simulink model "file2"  (R2025b)
settings: Solver=VariableStepAuto  StartTime=0.0  StopTime=1.0  RelTol=1e-3
InitFcn:
  | Voc= 32.9;
  | Iscn = 8.21;
  | K=1.38e-23;
  | N5=54;
  | Np=1;
  | G1 = 1000;
  | G2 = 859;
  | G3 = 659;
  | Gn = 1000;
  | Kv= - 0.123;
  | K1=0.0032;
  | T=301;
  | Tn = 300;
  | q=1.6e-19;
  | I0n = 9.58e-8;
  | Eg =1.12;
  | Ign =8.214;
  | Rs = 0.221;
  | Rp =414.5;
  | a=1.0;
libraries: spsVoltageMeasurementLib x7, spsSeriesRLCBranchLib x6, spsDiodeLib x3, spsControlledCurrentSourceLib x3, spsControlledVoltageSourceLib x1, spsCurrentMeasurementLib x1, simulink x1, spspowerguiLib x1
settings Model: Creator=cdsl09  LastModifiedBy=hp

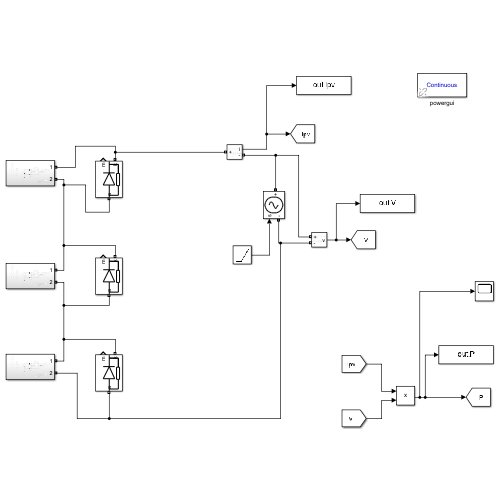
[thumbnail: Simulink's stored preview of the top-level diagram]
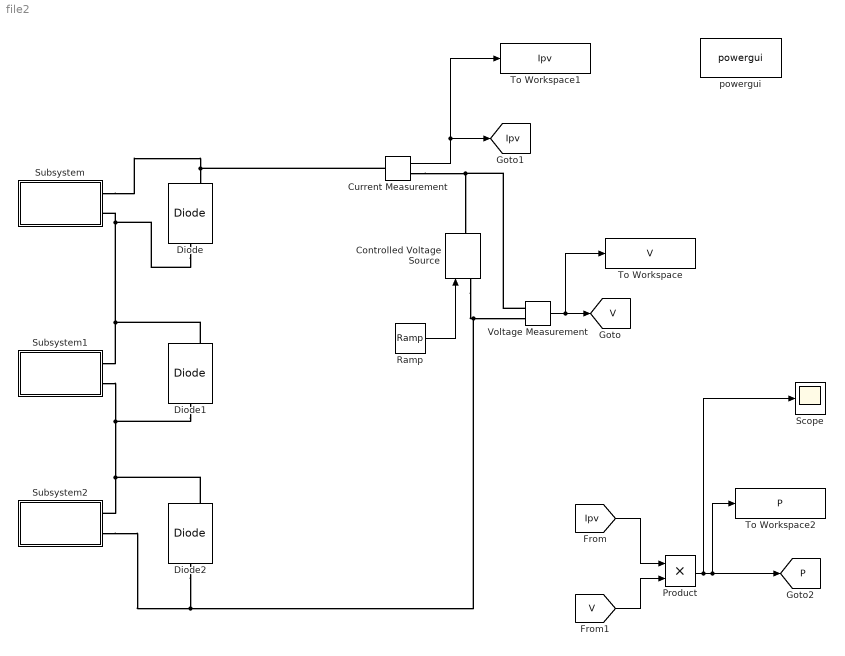
== system file2 ==
  Controlled Voltage Source : spsControlledVoltageSourceLib/Controlled Voltage Source  Initialize=on  Source_Type=AC  Amplitude=0  Phase=0  Frequency=0  Measurements=None
  Current Measurement : spsCurrentMeasurementLib/Current Measurement  PhasorSimulation=off  OutputType=Complex  PSBequivalent=0
  Diode : spsDiodeLib/Diode  Ron=0.001  Lon=0  Vf=0.8  IC=0  UseSnubber=0  Rs=500  Cs=250e-9  Measurements=on
  Diode1 : spsDiodeLib/Diode  Ron=0.001  Lon=0  Vf=0.8  IC=0  UseSnubber=0  Rs=500  Cs=250e-9  Measurements=on
  Diode2 : spsDiodeLib/Diode  Ron=0.001  Lon=0  Vf=0.8  IC=0  UseSnubber=0  Rs=500  Cs=250e-9  Measurements=on
  Product : Product
  Ramp : simulink/Sources/Ramp  slope=100  start=0  InitialOutput=0
  Scope : Scope
      settings: ActiveDisplayYMinimum=-293.34579  ActiveDisplayYMaximum=493.69358
  Subsystem : Subsystem
  Subsystem1 : Subsystem
  Subsystem2 : Subsystem
  To Workspace : ToWorkspace  VariableName=V  SampleTime=-1
  To Workspace1 : ToWorkspace  VariableName=Ipv  SampleTime=-1
  To Workspace2 : ToWorkspace  VariableName=P  SampleTime=-1
  Voltage Measurement : spsVoltageMeasurementLib/Voltage Measurement  PhasorSimulation=off  OutputType=Complex  PSBequivalent=0
  powergui : spspowerguiLib/powergui  Priority=1  SimulationMode=Continuous  SampleTime=50e-6  frequency=60  Iterations=50  frequencyindice=0  Pbase=100e6  ErrMax=1e-4  UnitsV=kV  UnitsW=MW  buscounter=0  FunctionMessages=off  echomessages=off  EnableUseOfTLC=off  CurrentSourceSwitches=off  DisableSnubberDevices=off  DisableRonSwitches=off  DisableVfSwitches=off  DisplayEquations=off  AutomaticDiscreteSolvers=off  SolverType=Tustin/Backward Euler (TBE)  Interpol=off  ExternalGateDelay=off  methode=off  Ts=100  x0status=blocks  SPID=on  SwTol=0  HookPort=off  NonlinearTolerance=1e-4  nMaxIteration=100  ContinueOnMaxIteration=off  RestoreLinks=warning  ResistiveCurrentMeasurement=off  Frange=[0:2:500]  Ylog=off  Xlog=on  ShowGrid=off  save=off  variable=ZData  structure=0  ZoomFFT=off  StartTime=0.0  cycles=1  DisplayStyle=1  fundamental=60  FreqAxis=off  MaxFrequency=1000  frequencyindicesteady=1  RmsSteady=1  display=off
  tag scope: Ipv=global, P=global, V=global
  wires:
  Ramp/1 -> Controlled Voltage Source/1
  Voltage Measurement/1 -> To Workspace/1, [V]
  Current Measurement/1 -> To Workspace1/1, [Ipv]
  [Ipv] -> Product/1
  [V] -> Product/2
  Product/1 -> Scope/1, To Workspace2/1, [P]
  connections:
  Subsystem/LConn1 -- Current Measurement/LConn1 -- Diode/RConn1
  Subsystem1/LConn1 -- Diode1/RConn1 -- Diode/LConn1 -- Subsystem/LConn2
  Subsystem1/LConn2 -- Diode1/LConn1 -- Diode2/RConn1 -- Subsystem2/LConn1
  Current Measurement/RConn1 -- Voltage Measurement/LConn1 -- Controlled Voltage Source/RConn1
  Controlled Voltage Source/LConn1 -- Diode2/LConn1 -- Subsystem2/LConn2 -- Voltage Measurement/LConn2

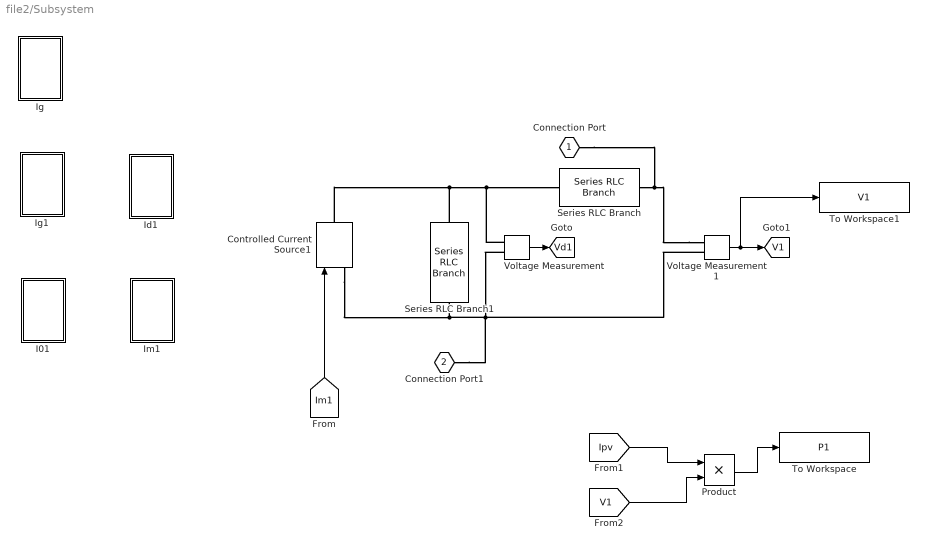
== system file2/Subsystem ==
  Controlled Current Source1 : spsControlledCurrentSourceLib/Controlled Current Source  Initialize=on  Source_Type=AC  Amplitude=0  Phase=0  Frequency=0  Measurements=None
  I01 : Subsystem
  Id1 : Subsystem
  Ig : Subsystem
  Ig1 : Subsystem
  Im1 : Subsystem
  Product : Product
  Series RLC Branch : spsSeriesRLCBranchLib/Series RLC Branch  LConnTagsString=__new0  RConnTagsString=__new0  BranchType=R  Resistance=Rs  Inductance=1e-3  SetiL0=off  InitialCurrent=0  Capacitance=1e-6  Setx0=off  InitialVoltage=0  Measurements=None
  Series RLC Branch1 : spsSeriesRLCBranchLib/Series RLC Branch  LConnTagsString=__new0  RConnTagsString=__new0  BranchType=R  Resistance=Rp  Inductance=1e-3  SetiL0=off  InitialCurrent=0  Capacitance=1e-6  Setx0=off  InitialVoltage=0  Measurements=None
  To Workspace : ToWorkspace  VariableName=P1  SaveFormat=Timeseries  SampleTime=-1
  To Workspace1 : ToWorkspace  VariableName=V1  SaveFormat=Timeseries  SampleTime=-1
  Voltage Measurement : spsVoltageMeasurementLib/Voltage Measurement  PhasorSimulation=off  OutputType=Complex  PSBequivalent=0
  Voltage Measurement1 : spsVoltageMeasurementLib/Voltage Measurement  PhasorSimulation=off  OutputType=Complex  PSBequivalent=0
  Connection Port : PMIOPort  Tag=simrfV2util1/Connection Port  Side=Left
  Connection Port1 : PMIOPort  Tag=simrfV2util1/Connection Port  Port=2  Side=Left
  tag scope: V1=global, Vd1=global
  wires:
  Product/1 -> To Workspace/1
  Voltage Measurement/1 -> [Vd1]
  Voltage Measurement1/1 -> To Workspace1/1, [V1]
  [Ipv] -> Product/1
  [Im1] -> Controlled Current Source1/1
  [V1] -> Product/2
  connections:
  Controlled Current Source1/LConn1 -- Connection Port1/RConn1 -- Voltage Measurement1/LConn2 -- Voltage Measurement/LConn2 -- Series RLC Branch1/LConn1
  Controlled Current Source1/RConn1 -- Series RLC Branch1/RConn1 -- Voltage Measurement/LConn1 -- Series RLC Branch/LConn1
  Voltage Measurement1/LConn1 -- Connection Port/RConn1 -- Series RLC Branch/RConn1

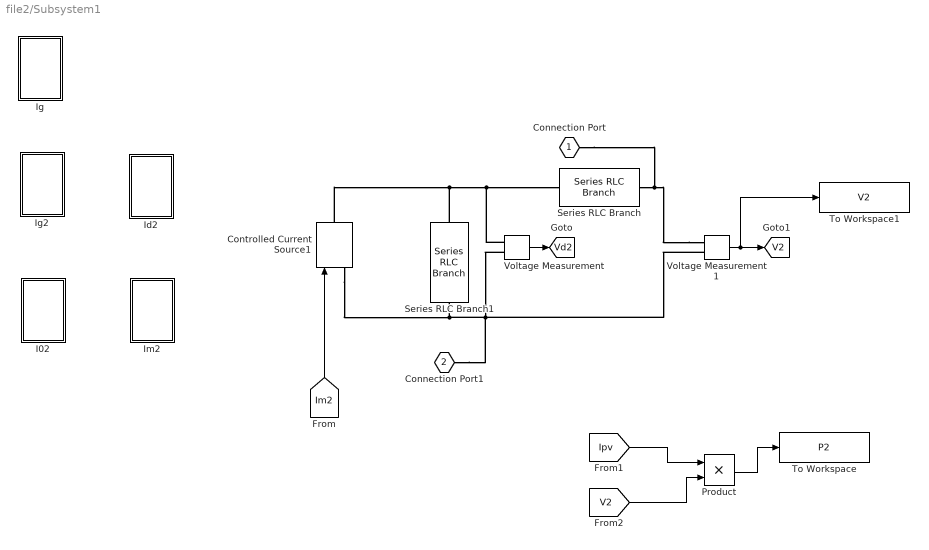
== system file2/Subsystem1 ==
  Controlled Current Source1 : spsControlledCurrentSourceLib/Controlled Current Source  Initialize=on  Source_Type=AC  Amplitude=0  Phase=0  Frequency=0  Measurements=None
  I02 : Subsystem
  Id2 : Subsystem
  Ig : Subsystem
  Ig2 : Subsystem
  Im2 : Subsystem
  Product : Product
  Series RLC Branch : spsSeriesRLCBranchLib/Series RLC Branch  LConnTagsString=__new0  RConnTagsString=__new0  BranchType=R  Resistance=Rs  Inductance=1e-3  SetiL0=off  InitialCurrent=0  Capacitance=1e-6  Setx0=off  InitialVoltage=0  Measurements=None
  Series RLC Branch1 : spsSeriesRLCBranchLib/Series RLC Branch  LConnTagsString=__new0  RConnTagsString=__new0  BranchType=R  Resistance=Rp  Inductance=1e-3  SetiL0=off  InitialCurrent=0  Capacitance=1e-6  Setx0=off  InitialVoltage=0  Measurements=None
  To Workspace : ToWorkspace  VariableName=P2  SaveFormat=Timeseries  SampleTime=-1
  To Workspace1 : ToWorkspace  VariableName=V2  SaveFormat=Timeseries  SampleTime=-1
  Voltage Measurement : spsVoltageMeasurementLib/Voltage Measurement  PhasorSimulation=off  OutputType=Complex  PSBequivalent=0
  Voltage Measurement1 : spsVoltageMeasurementLib/Voltage Measurement  PhasorSimulation=off  OutputType=Complex  PSBequivalent=0
  Connection Port : PMIOPort  Tag=simrfV2util1/Connection Port  Side=Left
  Connection Port1 : PMIOPort  Tag=simrfV2util1/Connection Port  Port=2  Side=Left
  tag scope: V2=global, Vd2=global
  wires:
  Product/1 -> To Workspace/1
  Voltage Measurement/1 -> [Vd2]
  Voltage Measurement1/1 -> To Workspace1/1, [V2]
  [Ipv] -> Product/1
  [Im2] -> Controlled Current Source1/1
  [V2] -> Product/2
  connections:
  Controlled Current Source1/LConn1 -- Series RLC Branch1/LConn1 -- Voltage Measurement1/LConn2 -- Voltage Measurement/LConn2 -- Connection Port1/RConn1
  Controlled Current Source1/RConn1 -- Series RLC Branch1/RConn1 -- Voltage Measurement/LConn1 -- Series RLC Branch/LConn1
  Voltage Measurement1/LConn1 -- Series RLC Branch/RConn1 -- Connection Port/RConn1

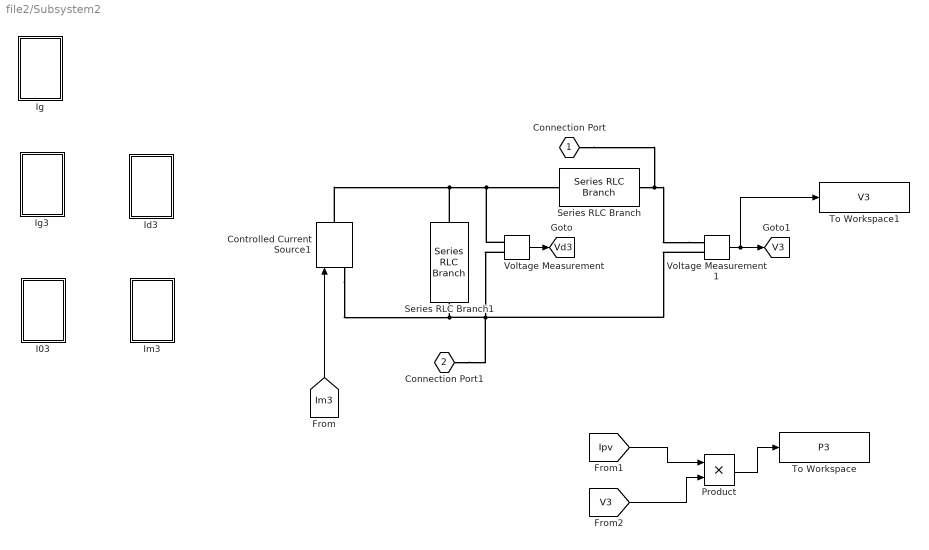
== system file2/Subsystem2 ==
  Controlled Current Source1 : spsControlledCurrentSourceLib/Controlled Current Source  Initialize=on  Source_Type=AC  Amplitude=0  Phase=0  Frequency=0  Measurements=None
  I03 : Subsystem
  Id3 : Subsystem
  Ig : Subsystem
  Ig3 : Subsystem
  Im3 : Subsystem
  Product : Product
  Series RLC Branch : spsSeriesRLCBranchLib/Series RLC Branch  LConnTagsString=__new0  RConnTagsString=__new0  BranchType=R  Resistance=Rs  Inductance=1e-3  SetiL0=off  InitialCurrent=0  Capacitance=1e-6  Setx0=off  InitialVoltage=0  Measurements=None
  Series RLC Branch1 : spsSeriesRLCBranchLib/Series RLC Branch  LConnTagsString=__new0  RConnTagsString=__new0  BranchType=R  Resistance=Rp  Inductance=1e-3  SetiL0=off  InitialCurrent=0  Capacitance=1e-6  Setx0=off  InitialVoltage=0  Measurements=None
  To Workspace : ToWorkspace  VariableName=P3  SaveFormat=Timeseries  SampleTime=-1
  To Workspace1 : ToWorkspace  VariableName=V3  SaveFormat=Timeseries  SampleTime=-1
  Voltage Measurement : spsVoltageMeasurementLib/Voltage Measurement  PhasorSimulation=off  OutputType=Complex  PSBequivalent=0
  Voltage Measurement1 : spsVoltageMeasurementLib/Voltage Measurement  PhasorSimulation=off  OutputType=Complex  PSBequivalent=0
  Connection Port : PMIOPort  Tag=simrfV2util1/Connection Port  Side=Left
  Connection Port1 : PMIOPort  Tag=simrfV2util1/Connection Port  Port=2  Side=Left
  tag scope: V3=global, Vd3=global
  wires:
  Product/1 -> To Workspace/1
  Voltage Measurement/1 -> [Vd3]
  Voltage Measurement1/1 -> To Workspace1/1, [V3]
  [Ipv] -> Product/1
  [Im3] -> Controlled Current Source1/1
  [V3] -> Product/2
  connections:
  Controlled Current Source1/LConn1 -- Series RLC Branch1/LConn1 -- Voltage Measurement1/LConn2 -- Voltage Measurement/LConn2 -- Connection Port1/RConn1
  Controlled Current Source1/RConn1 -- Series RLC Branch1/RConn1 -- Voltage Measurement/LConn1 -- Series RLC Branch/LConn1
  Voltage Measurement1/LConn1 -- Series RLC Branch/RConn1 -- Connection Port/RConn1

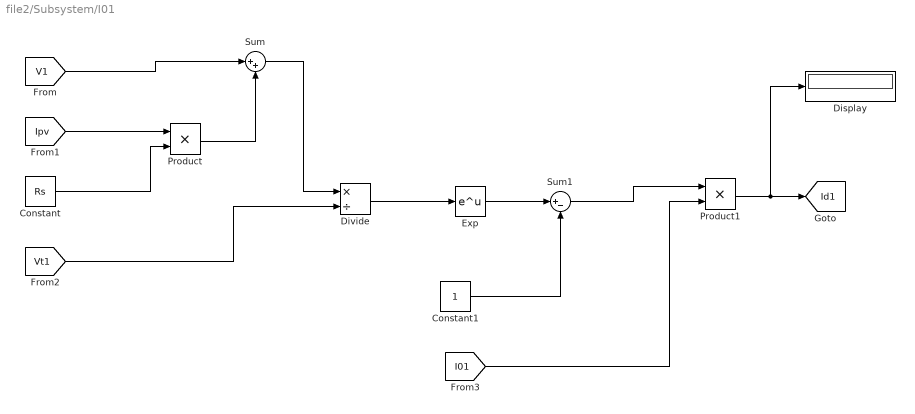
== system file2/Subsystem/I01 ==
  Constant : Constant  Value=Rs
  Constant1 : Constant
  Display : Display
  Divide : Product  Inputs=*/
  Exp : Math
  Product : Product
  Product1 : Product
  Sum : Sum  Inputs=|++
  Sum1 : Sum  Inputs=|+-
  tag scope: Id1=global
  wires:
  Exp/1 -> Sum1/1
  Divide/1 -> Exp/1
  [I01] -> Product1/2
  Sum/1 -> Divide/1
  [V1] -> Sum/1
  Product/1 -> Sum/2
  Constant1/1 -> Sum1/2
  Sum1/1 -> Product1/1
  Constant/1 -> Product/2
  [Ipv] -> Product/1
  [Vt1] -> Divide/2
  Product1/1 -> Display/1, [Id1]

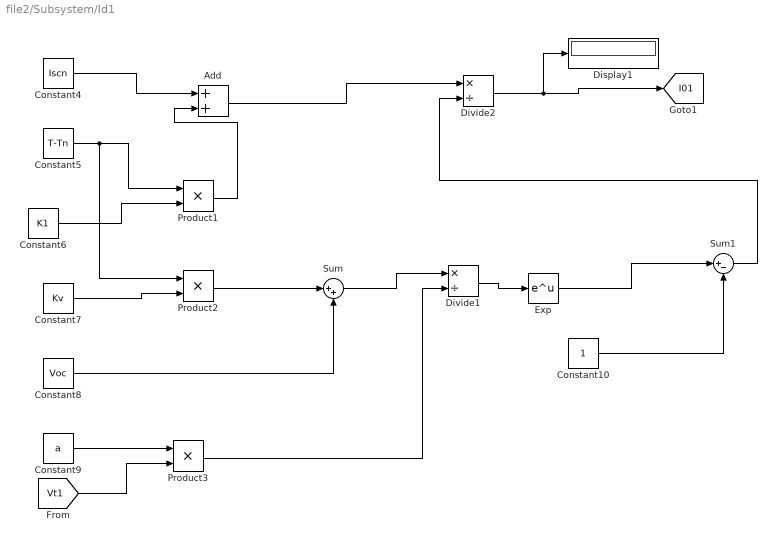
== system file2/Subsystem/Id1 ==
  Add : Sum
  Constant10 : Constant
  Constant4 : Constant  Value=Iscn
  Constant5 : Constant  Value=T-Tn
  Constant6 : Constant  Value=K1
  Constant7 : Constant  Value=Kv
  Constant8 : Constant  Value=Voc
  Constant9 : Constant  Value=a
  Display1 : Display
  Divide1 : Product  Inputs=*/
  Divide2 : Product  Inputs=*/
  Exp : Math
  Product1 : Product
  Product2 : Product
  Product3 : Product
  Sum : Sum  Inputs=|++
  Sum1 : Sum  Inputs=|+-
  tag scope: I01=global
  wires:
  Product2/1 -> Sum/1
  Constant8/1 -> Sum/2
  Constant4/1 -> Add/1
  Constant5/1 -> Product2/1, Product1/1
  Product1/1 -> Add/2
  Product3/1 -> Divide1/2
  Divide1/1 -> Exp/1
  Constant6/1 -> Product1/2
  Sum1/1 -> Divide2/2
  [Vt1] -> Product3/2
  Constant9/1 -> Product3/1
  Divide2/1 -> Display1/1, [I01]
  Constant10/1 -> Sum1/2
  Add/1 -> Divide2/1
  Constant7/1 -> Product2/2
  Exp/1 -> Sum1/1
  Sum/1 -> Divide1/1

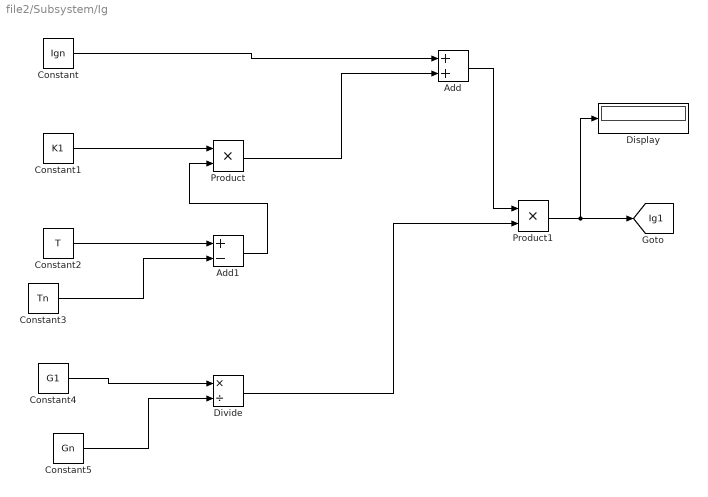
== system file2/Subsystem/Ig ==
  Add : Sum
  Add1 : Sum  Inputs=+-
  Constant : Constant  Value=Ign
  Constant1 : Constant  Value=K1
  Constant2 : Constant  Value=T
  Constant3 : Constant  Value=Tn
  Constant4 : Constant  Value=G1  VectorParams1D=off
  Constant5 : Constant  Value=Gn
  Display : Display
  Divide : Product  Inputs=*/
  Product : Product
  Product1 : Product
  tag scope: Ig1=global
  wires:
  Product1/1 -> Display/1, [Ig1]
  Constant3/1 -> Add1/2
  Constant5/1 -> Divide/2
  Add1/1 -> Product/2
  Constant4/1 -> Divide/1
  Product/1 -> Add/2
  Constant2/1 -> Add1/1
  Add/1 -> Product1/1
  Constant1/1 -> Product/1
  Constant/1 -> Add/1
  Divide/1 -> Product1/2

== system file2/Subsystem/Ig1 ==
  Constant : Constant  Value=N5
  Constant1 : Constant  Value=K
  Constant2 : Constant  Value=T
  Constant3 : Constant  Value=q
  Display : Display
  Divide : Product  Inputs=*/
  Product : Product  Inputs=3
  tag scope: Vt1=global
  wires:
  Product/1 -> Divide/1
  Constant/1 -> Product/1
  Constant3/1 -> Divide/2
  Constant1/1 -> Product/2
  Constant2/1 -> Product/3
  Divide/1 -> Display/1, [Vt1]

== system file2/Subsystem/Im1 ==
  Add : Sum  Inputs=+-
  Display : Display
  tag scope: Im1=global
  wires:
  [Ig1] -> Add/1
  [Id1] -> Add/2
  Add/1 -> Display/1, [Im1]

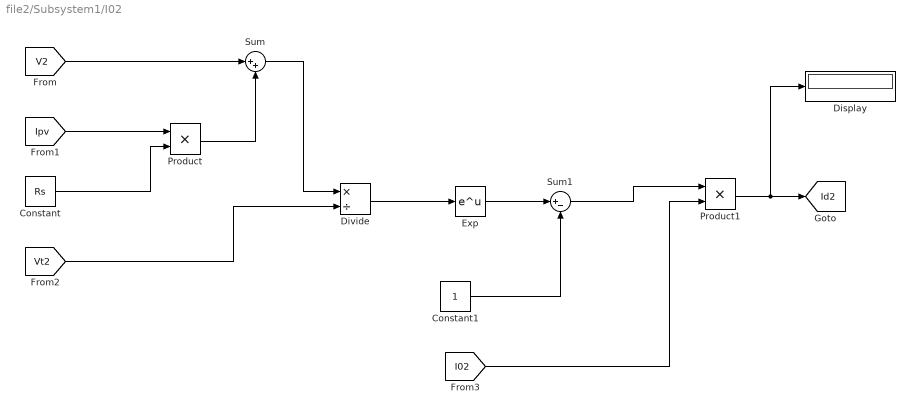
== system file2/Subsystem1/I02 ==
  Constant : Constant  Value=Rs
  Constant1 : Constant
  Display : Display
  Divide : Product  Inputs=*/
  Exp : Math
  Product : Product
  Product1 : Product
  Sum : Sum  Inputs=|++
  Sum1 : Sum  Inputs=|+-
  tag scope: Id2=global
  wires:
  Exp/1 -> Sum1/1
  Divide/1 -> Exp/1
  [I02] -> Product1/2
  Sum/1 -> Divide/1
  [V2] -> Sum/1
  Product/1 -> Sum/2
  Constant1/1 -> Sum1/2
  Sum1/1 -> Product1/1
  Constant/1 -> Product/2
  [Ipv] -> Product/1
  [Vt2] -> Divide/2
  Product1/1 -> Display/1, [Id2]

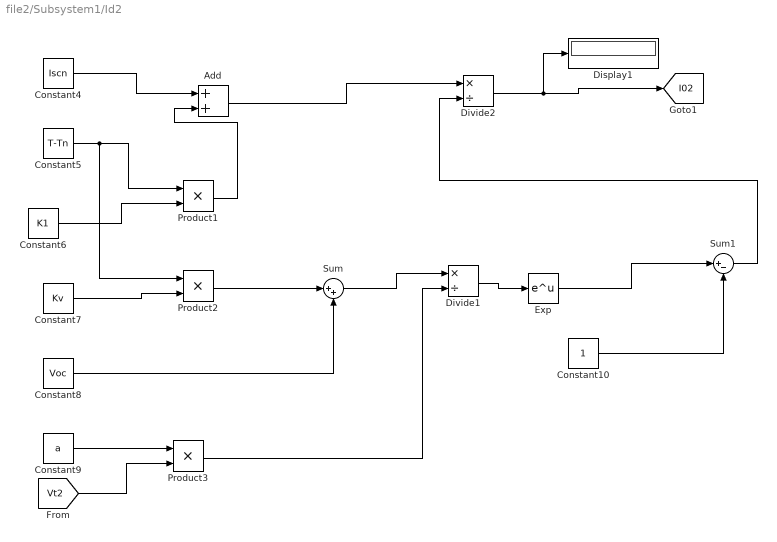
== system file2/Subsystem1/Id2 ==
  Add : Sum
  Constant10 : Constant
  Constant4 : Constant  Value=Iscn
  Constant5 : Constant  Value=T-Tn
  Constant6 : Constant  Value=K1
  Constant7 : Constant  Value=Kv
  Constant8 : Constant  Value=Voc
  Constant9 : Constant  Value=a
  Display1 : Display
  Divide1 : Product  Inputs=*/
  Divide2 : Product  Inputs=*/
  Exp : Math
  Product1 : Product
  Product2 : Product
  Product3 : Product
  Sum : Sum  Inputs=|++
  Sum1 : Sum  Inputs=|+-
  tag scope: I02=global
  wires:
  Product2/1 -> Sum/1
  Constant8/1 -> Sum/2
  Constant4/1 -> Add/1
  Constant5/1 -> Product2/1, Product1/1
  Product1/1 -> Add/2
  Product3/1 -> Divide1/2
  Divide1/1 -> Exp/1
  Constant6/1 -> Product1/2
  Sum1/1 -> Divide2/2
  [Vt2] -> Product3/2
  Constant9/1 -> Product3/1
  Divide2/1 -> Display1/1, [I02]
  Constant10/1 -> Sum1/2
  Add/1 -> Divide2/1
  Constant7/1 -> Product2/2
  Exp/1 -> Sum1/1
  Sum/1 -> Divide1/1

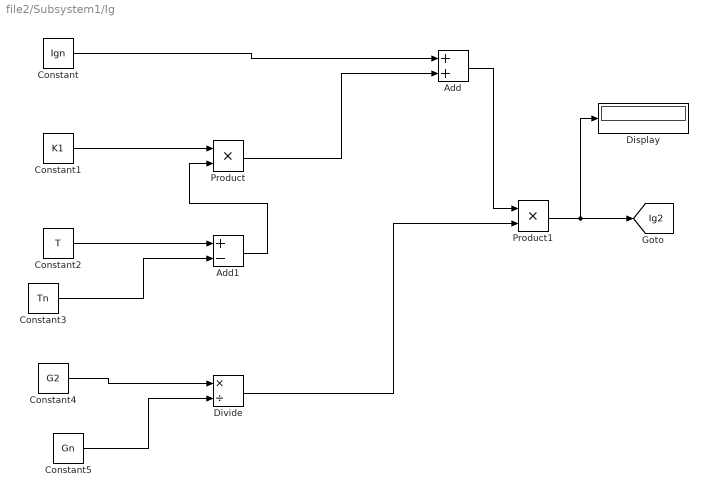
== system file2/Subsystem1/Ig ==
  Add : Sum
  Add1 : Sum  Inputs=+-
  Constant : Constant  Value=Ign
  Constant1 : Constant  Value=K1
  Constant2 : Constant  Value=T
  Constant3 : Constant  Value=Tn
  Constant4 : Constant  Value=G2  VectorParams1D=off
  Constant5 : Constant  Value=Gn
  Display : Display
  Divide : Product  Inputs=*/
  Product : Product
  Product1 : Product
  tag scope: Ig2=global
  wires:
  Product1/1 -> Display/1, [Ig2]
  Constant3/1 -> Add1/2
  Constant5/1 -> Divide/2
  Add1/1 -> Product/2
  Constant4/1 -> Divide/1
  Product/1 -> Add/2
  Constant2/1 -> Add1/1
  Add/1 -> Product1/1
  Constant1/1 -> Product/1
  Constant/1 -> Add/1
  Divide/1 -> Product1/2

== system file2/Subsystem1/Ig2 ==
  Constant : Constant  Value=N5
  Constant1 : Constant  Value=K
  Constant2 : Constant  Value=T
  Constant3 : Constant  Value=q
  Display : Display
  Divide : Product  Inputs=*/
  Product : Product  Inputs=3
  tag scope: Vt2=global
  wires:
  Product/1 -> Divide/1
  Constant/1 -> Product/1
  Constant3/1 -> Divide/2
  Constant1/1 -> Product/2
  Constant2/1 -> Product/3
  Divide/1 -> Display/1, [Vt2]

== system file2/Subsystem1/Im2 ==
  Add : Sum  Inputs=+-
  Display : Display
  tag scope: Im2=global
  wires:
  [Ig2] -> Add/1
  [Id2] -> Add/2
  Add/1 -> Display/1, [Im2]

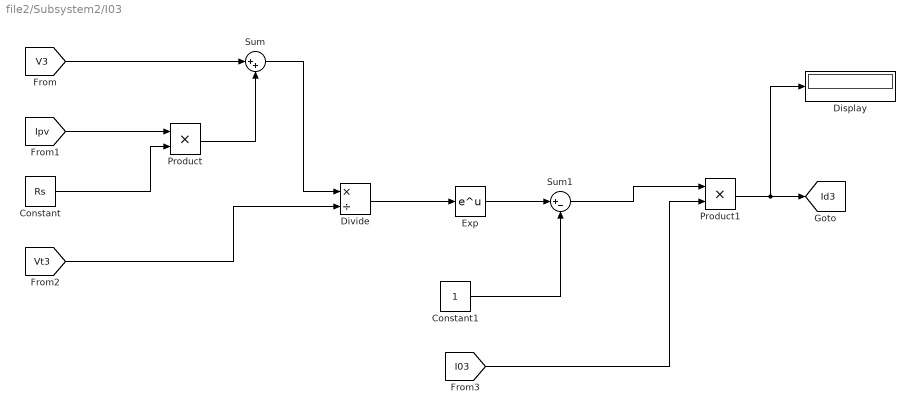
== system file2/Subsystem2/I03 ==
  Constant : Constant  Value=Rs
  Constant1 : Constant
  Display : Display
  Divide : Product  Inputs=*/
  Exp : Math
  Product : Product
  Product1 : Product
  Sum : Sum  Inputs=|++
  Sum1 : Sum  Inputs=|+-
  tag scope: Id3=global
  wires:
  Exp/1 -> Sum1/1
  Divide/1 -> Exp/1
  [I03] -> Product1/2
  Sum/1 -> Divide/1
  [V3] -> Sum/1
  Product/1 -> Sum/2
  Constant1/1 -> Sum1/2
  Sum1/1 -> Product1/1
  Constant/1 -> Product/2
  [Ipv] -> Product/1
  [Vt3] -> Divide/2
  Product1/1 -> Display/1, [Id3]

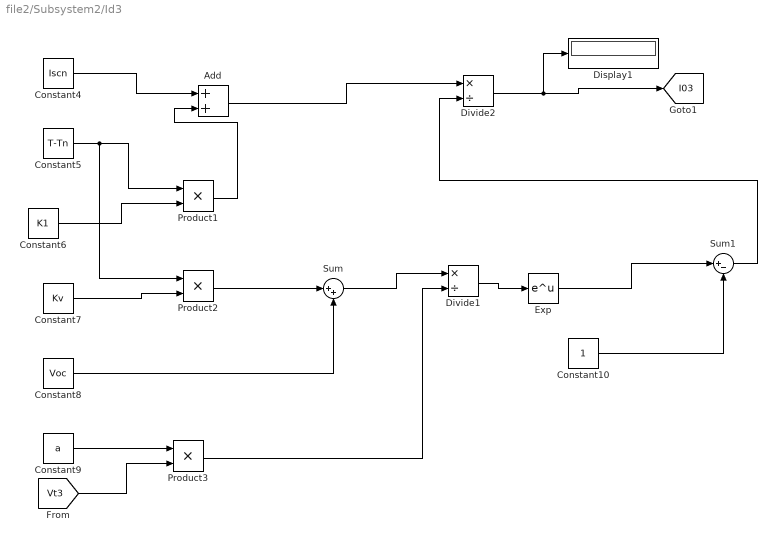
== system file2/Subsystem2/Id3 ==
  Add : Sum
  Constant10 : Constant
  Constant4 : Constant  Value=Iscn
  Constant5 : Constant  Value=T-Tn
  Constant6 : Constant  Value=K1
  Constant7 : Constant  Value=Kv
  Constant8 : Constant  Value=Voc
  Constant9 : Constant  Value=a
  Display1 : Display
  Divide1 : Product  Inputs=*/
  Divide2 : Product  Inputs=*/
  Exp : Math
  Product1 : Product
  Product2 : Product
  Product3 : Product
  Sum : Sum  Inputs=|++
  Sum1 : Sum  Inputs=|+-
  tag scope: I03=global
  wires:
  Product2/1 -> Sum/1
  Constant8/1 -> Sum/2
  Constant4/1 -> Add/1
  Constant5/1 -> Product2/1, Product1/1
  Product1/1 -> Add/2
  Product3/1 -> Divide1/2
  Divide1/1 -> Exp/1
  Constant6/1 -> Product1/2
  Sum1/1 -> Divide2/2
  [Vt3] -> Product3/2
  Constant9/1 -> Product3/1
  Divide2/1 -> Display1/1, [I03]
  Constant10/1 -> Sum1/2
  Add/1 -> Divide2/1
  Constant7/1 -> Product2/2
  Exp/1 -> Sum1/1
  Sum/1 -> Divide1/1

== system file2/Subsystem2/Ig ==
  Add : Sum
  Add1 : Sum  Inputs=+-
  Constant : Constant  Value=Ign
  Constant1 : Constant  Value=K1
  Constant2 : Constant  Value=T
  Constant3 : Constant  Value=Tn
  Constant4 : Constant  Value=G3  VectorParams1D=off
  Constant5 : Constant  Value=Gn
  Display : Display
  Divide : Product  Inputs=*/
  Product : Product
  Product1 : Product
  tag scope: Ig3=global
  wires:
  Product1/1 -> Display/1, [Ig3]
  Constant3/1 -> Add1/2
  Constant5/1 -> Divide/2
  Add1/1 -> Product/2
  Constant4/1 -> Divide/1
  Product/1 -> Add/2
  Constant2/1 -> Add1/1
  Add/1 -> Product1/1
  Constant1/1 -> Product/1
  Constant/1 -> Add/1
  Divide/1 -> Product1/2

== system file2/Subsystem2/Ig3 ==
  Constant : Constant  Value=N5
  Constant1 : Constant  Value=K
  Constant2 : Constant  Value=T
  Constant3 : Constant  Value=q
  Display : Display
  Divide : Product  Inputs=*/
  Product : Product  Inputs=3
  tag scope: Vt3=global
  wires:
  Product/1 -> Divide/1
  Constant/1 -> Product/1
  Constant3/1 -> Divide/2
  Constant1/1 -> Product/2
  Constant2/1 -> Product/3
  Divide/1 -> Display/1, [Vt3]

== system file2/Subsystem2/Im3 ==
  Add : Sum  Inputs=+-
  Display : Display
  tag scope: Im3=global
  wires:
  [Ig3] -> Add/1
  [Id3] -> Add/2
  Add/1 -> Display/1, [Im3]
